simulink model "DC_motor_simulink"  (R2015b)
settings: Solver=VariableStepAuto  SolverMode=SingleTasking  StartTime=0.0  StopTime=15  RelTol=1e-12
values from neighbouring files (symbols this model uses):
  A = [0   1 ... (first row only)    [DC_motor_example_LQR_v2.m]    (also in First_example_LQR.m = 1; IP.m = [0     0     1      0; ip_example.m = [ 0          0        1         0; suspension_estimator.m = [      0            1           0           0)
  B = [0 ... (first row only)    [DC_motor_example_LQR_v2.m]    (also in First_example_LQR.m = 1; IP.m = [0; 0; 3.7778; -12.3862]; ip_example.m = [ 0; suspension_estimator.m = [ 0)
  K = lqr(A,B,Q,R)    [DC_motor_example_LQR_v2.m]    (also in First_example_LQR.m = K_vector(j); ip_example.m = acker(A,B,cl_poles); suspension_estimator.m = acker(A,B,cl_poles); two_tanks_tracking_controller.m = place(A,B,cl_poles))
settings Model: Creator=magudelo  LastModifiedBy=Mauricio
settings DataIOCC: LimitDataPoints=off  ReturnWorkspaceOutputs=on
settings DebuggingCC: AllowSymbolicDim=on  SFUnexpectedBacktrackingDiag=error  SFNoUnconditionalDefaultTransitionDiag=error
settings ModelReferenceCC: PropagateSignalLabelsOutOfModel=on
settings SFSimCC: SimUseLocalCustomCode=on
settings RTWCC: RTWUseLocalCustomCode=on
settings GRTTargetCC: TargetLangStandard=C99 (ISO)
settings ConfigComp: CovMetricSettings=dwe  CovHtmlReporting=off  CovSaveCumulativeToWorkspaceVar=off  CovSaveSingleToWorkspaceVar=off  CovModelRefEnable=Off  CovExternalEMLEnable=on

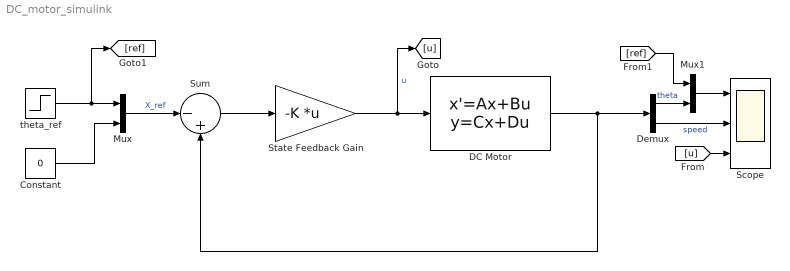
== system DC_motor_simulink ==
  Constant : Constant  Value=0
  DC Motor : StateSpace  A=A  B=B  C=eye(2,2)  D=zeros(2,1)  X0=0
  Demux : Demux  Outputs=2
  Mux : Mux  Inputs=2
  Mux1 : Mux  Inputs=2
  Scope : Scope  NumInputPorts=3
  State Feedback Gain : Gain  Gain=-K  Multiplication=Matrix(K*u)
  Sum : Sum  Inputs=|-+
  theta_ref : Step  SampleTime=0
  wires:
  Mux/1 -> Sum/1  "X_ref"
  Constant/1 -> Mux/2
  theta_ref/1 -> [ref], Mux/1
  Sum/1 -> State Feedback Gain/1
  State Feedback Gain/1 -> [u], DC Motor/1  "u"
  Demux/1 -> Mux1/2  "theta"
  Mux1/1 -> Scope/1
  Demux/2 -> Scope/2  "speed"
  [u] -> Scope/3
  [ref] -> Mux1/1
  DC Motor/1 -> Demux/1, Sum/2
